simulink model "zadanie_1"  (Simulink 7.7)
settings: Solver=ode4  StartTime=0.0  StopTime=50.0  FixedStep=0.01  RelTol=1e-3
settings Model: Creator=Aleksander  LastModifiedBy=Jacek
settings DataIOCC: LimitDataPoints=off  SignalLoggingSaveFormat=Dataset
settings OptimizationCC: ExpressionDepthLimit=128
settings CodeAppCC: CustomSymbolStrType=$N$R$M_T
settings GRTTargetCC: CombineOutputUpdateFcns=on

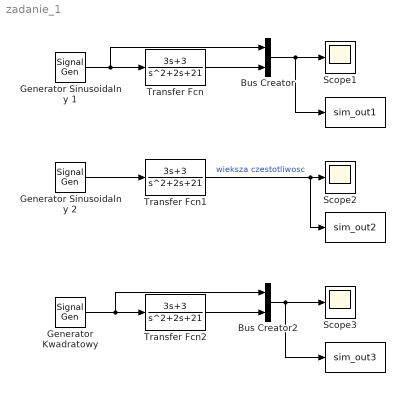
== system zadanie_1 ==
  " " : ToWorkspace  VariableName=sim_out1  SampleTime=-1  SaveFormat=Array
  "   " : ToWorkspace  VariableName=sim_out2  SampleTime=-1  SaveFormat=Array
  "       " : ToWorkspace  VariableName=sim_out3  SampleTime=-1  SaveFormat=Array
  Bus Creator : BusCreator  Inputs=2
  Bus Creator2 : BusCreator  Inputs=2
  Generator Kwadratowy : SignalGenerator  WaveForm=square  Frequency=0.04
  Generator Sinusoidalny 1 : SignalGenerator  Frequency=0.1
  Generator Sinusoidalny 2 : SignalGenerator  Amplitude=3  Frequency=2
  Scope1 : Scope
      settings: TimeRange=50  YMin=-1.5  YMax=1.5  SaveName=ScopeData3
  Scope2 : Scope
      settings: TimeRange=50  YMin=-1.5  YMax=1.5
  Scope3 : Scope
      settings: TimeRange=50  YMin=-1.5  YMax=1.5
  Transfer Fcn : TransferFcn  Numerator=[3 3]  Denominator=[1 2 21]
  Transfer Fcn1 : TransferFcn  Numerator=[3 3]  Denominator=[1 2 21]
  Transfer Fcn2 : TransferFcn  Numerator=[3 3]  Denominator=[1 2 21]
  wires:
  Generator Sinusoidalny 2/1 -> Transfer Fcn1/1
  Generator Kwadratowy/1 -> Transfer Fcn2/1, Bus Creator2/1
  Generator Sinusoidalny 1/1 -> Transfer Fcn/1, Bus Creator/1
  Bus Creator/1 -> Scope1/1, " "/1
  Bus Creator2/1 -> Scope3/1, "       "/1
  Transfer Fcn/1 -> Bus Creator/2
  Transfer Fcn2/1 -> Bus Creator2/2
  Transfer Fcn1/1 -> Scope2/1, "   "/1  "wieksza czestotliwosc"
